simulink model "ISStelerobotics"  (R2022b)
settings: Solver=VariableStepAuto  StartTime=0.0  StopTime=10  RelTol=1e-3
InitFcn:
  | gammaM = [1 0 0; 0 1 0; 0 0 1];
  | gammaS = [1 0 0; 0 1 0; 0 0 1];
  | Km = 300.*[1 0 0; 0 1 0; 0 0 1];
  | Ks = 300.*[1 0 0; 0 1 0; 0 0 1];
settings Model: Creator=negin  LastModifiedBy=Administrator
settings DebuggingCC: UnconnectedInputMsg=warning  UnconnectedOutputMsg=warning  UnconnectedLineMsg=warning
settings ModelReferenceCC: EnableRefExpFcnMdlSchedulingChecks=on
settings RTWCC: DLArmComputeVersion=19.05

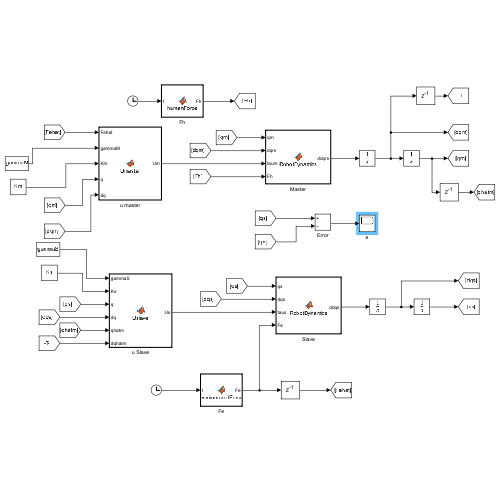
[thumbnail: Simulink's stored preview of the top-level diagram]
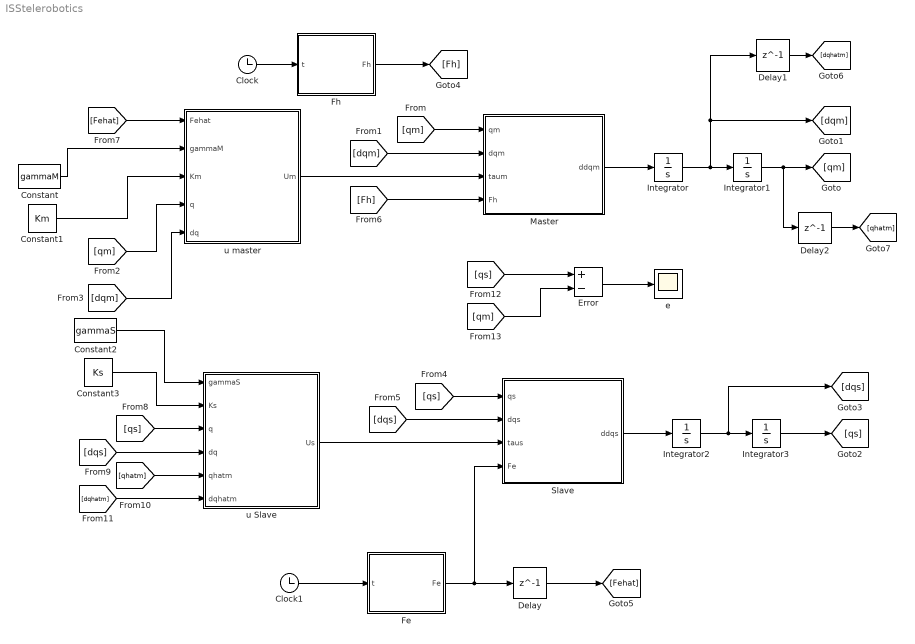
== system ISStelerobotics ==
  Clock : Clock
  Clock1 : Clock
  Constant : Constant  Value=gammaM  VectorParams1D=off
  Constant1 : Constant  Value=Km  VectorParams1D=off
  Constant2 : Constant  Value=gammaS  VectorParams1D=off
  Constant3 : Constant  Value=Ks  VectorParams1D=off
  Delay : Delay  DelayLength=1  InitialCondition=0
  Delay1 : Delay  DelayLength=1  InitialCondition=0
  Delay2 : Delay  DelayLength=1  InitialCondition=0
  Error : Sum  Inputs=+-
  Fe : MATLAB Function  TreatAsAtomicUnit=on
  Fh : MATLAB Function  TreatAsAtomicUnit=on
  Integrator{,1..3} (4 alike) : Integrator  InitialCondition=[0; 0; 0]
  Master : MATLAB Function  TreatAsAtomicUnit=on
  Slave : MATLAB Function  TreatAsAtomicUnit=on
  e : Scope
  u Slave : MATLAB Function  TreatAsAtomicUnit=on
  u master : MATLAB Function  TreatAsAtomicUnit=on
  wires:
  Clock/1 -> Fh/1(t)
  Fh/1(Fh) -> [Fh]
  u master/1(Um) -> Master/3(taum)
  Master/1(ddqm) -> Integrator/1
  Integrator/1 -> Delay1/1, [dqm], Integrator1/1
  Integrator1/1 -> Delay2/1, [qm]
  [qm] -> Master/1(qm)
  [dqm] -> Master/2(dqm)
  Constant/1 -> u master/2(gammaM)
  Constant1/1 -> u master/3(Km)
  [qm] -> u master/4(q)
  [dqm] -> u master/5(dq)
  Slave/1(ddqs) -> Integrator2/1
  Integrator2/1 -> [dqs], Integrator3/1
  Integrator3/1 -> [qs]
  [dqs] -> Slave/2(dqs)
  [qs] -> Slave/1(qs)
  u Slave/1(Us) -> Slave/3(taus)
  [Fh] -> Master/4(Fh)
  Clock1/1 -> Fe/1(t)
  Fe/1(Fe) -> Delay/1, Slave/4(Fe)
  Delay/1 -> [Fehat]
  [Fehat] -> u master/1(Fehat)
  Constant2/1 -> u Slave/1(gammaS)
  Constant3/1 -> u Slave/2(Ks)
  [qs] -> u Slave/3(q)
  [dqs] -> u Slave/4(dq)
  [dqhatm] -> u Slave/6(dqhatm)
  [qhatm] -> u Slave/5(qhatm)
  Delay1/1 -> [dqhatm]
  Delay2/1 -> [qhatm]
  [qs] -> Error/1
  [qm] -> Error/2
  Error/1 -> e/1

== matlab function ISStelerobotics/Master ==
  data: qm input; ddqm output; dqm input; taum input; Fh input
function ddqm = RobotDynamics(qm, dqm, taum, Fh)

m1 = 1;
m2 = 1;
m3 = 1;

l1 = 1;
l2 = 1;
l3 = 1;

r1 = l1/2;
r2 = l2/2;
r3 = l3/2;

R1 = 0.05;
R2 = 0.05;
R3 = 0.05;

g = 9.81;

a1 = m2*r2^2 + m3*l2^2;
a2 = m3*r3^2;
a3 = m3*r3*l2;
b1 = (m2*r2 + m3*l2)*g;
b2 = m3*r3*g;
I1 = 0.5*m1*R1^2;
I2 = 0.5*m2*R2^2;
I3 = 0.5*m3*R3^2;

M11 = a1*cos(qm(2))^2 + a2*cos(qm(2) + qm(3))^2 + 2*a3*cos(qm(2))*cos(qm(2) + qm(3)) + I1;
M12 = 0; 
M13 = 0; 
M21 = 0; 
M31 = 0;
M22 = a1 + a2 + 2*a3*cos(qm(3)) + I2;
M23 = a2 + a3*cos(qm(3));
M32 = a2 + a3*cos(qm(3));
M33 = a2 + I3;
M = [M11 M12 M13; M21 M22 M23; M31 M32 M33];

C11 = -0.5*a1*dqm(2)*sin(2*qm(2)) - 0.5*a2*(dqm(2) + dqm(3))*sin(2*qm(2) + 2*qm(3))...
    - a3*dqm(2)*sin(2*qm(2) + qm(3)) - a3*dqm(3)*cos(qm(2))*sin(qm(2) + qm(3));
C12 = -0.5*a1*dqm(1)*sin(2*qm(2)) - 0.5*a2*dqm(1)*sin(2*qm(2) + 2*qm(3)) - ...
    a3*dqm(1)*sin(2*qm(2) + qm(3));
C13 = -0.5*a2*dqm(1)*sin(2*qm(2) + 2*qm(3)) - a3*dqm(1)*cos(qm(2))*sin(qm(2) + qm(3));
C21 = -C12;
C22 = -a3*dqm(3)*sin(qm(3));
C23 = -a3*(dqm(2) + dqm(3))*sin(qm(3));
C31 = -C13;
C32 = a3*dqm(2)*sin(qm(3));
C33 = 0;
C = [C11 C12 C13; C21 C22 C23; C31 C32 C33];

G11 = 0;
G21 = m2*l2*sin(qm(2))*g/2 - m3*l3*sin(qm(2) + qm(3))*g/2 - m3*l2*sin(qm(2))*g;
G31 = -m3*l3*sin(qm(2) + qm(3))*g/2;
G = [G11; G21; G31];

ddqm = inv(M)*(taum + Fh - C*dqm - G);
end

== matlab function ISStelerobotics/Fh ==
  data: t input; Fh output
function Fh = humanForce(t)

Fh = [t; 2*t; 3*t];

end

== matlab function ISStelerobotics/u master ==
  data: Fehat input; Um output; gammaM input; Km input; q input; dq input
function Um = Umaster(Fehat, gammaM, Km, q, dq)

m1 = 1;
m2 = 1;
m3 = 1;

l1 = 1;
l2 = 1;
l3 = 1;

r1 = l1/2;
r2 = l2/2;
r3 = l3/2;

R1 = 0.05;
R2 = 0.05;
R3 = 0.05;

g = 9.81;

a1 = m2*r2^2 + m3*l2^2;
a2 = m3*r3^2;
a3 = m3*r3*l2;
b1 = (m2*r2 + m3*l2)*g;
b2 = m3*r3*g;
I1 = 0.5*m1*R1^2;
I2 = 0.5*m2*R2^2;
I3 = 0.5*m3*R3^2;

M11 = a1*cos(q(2))^2 + a2*cos(q(2) + q(3))^2 + 2*a3*cos(q(2))*cos(q(2) + q(3)) + I1;
M12 = 0; 
M13 = 0; 
M21 = 0; 
M31 = 0;
M22 = a1 + a2 + 2*a3*cos(q(3)) + I2;
M23 = a2 + a3*cos(q(3));
M32 = a2 + a3*cos(q(3));
M33 = a2 + I3;
M = [M11 M12 M13; M21 M22 M23; M31 M32 M33];

C11 = -0.5*a1*dq(2)*sin(2*q(2)) - 0.5*a2*(dq(2) + dq(3))*sin(2*q(2) + 2*q(3))...
    - a3*dq(2)*sin(2*q(2) + q(3)) - a3*dq(3)*cos(q(2))*sin(q(2) + q(3));
C12 = -0.5*a1*dq(1)*sin(2*q(2)) - 0.5*a2*dq(1)*sin(2*q(2) + 2*q(3)) - ...
    a3*dq(1)*sin(2*q(2) + q(3));
C13 = -0.5*a2*dq(1)*sin(2*q(2) + 2*q(3)) - a3*dq(1)*cos(q(2))*sin(q(2) + q(3));
C21 = -C12;
C22 = -a3*dq(3)*sin(q(3));
C23 = -a3*(dq(2) + dq(3))*sin(q(3));
C31 = -C13;
C32 = a3*dq(2)*sin(q(3));
C33 = 0;
C = [C11 C12 C13; C21 C22 C23; C31 C32 C33];

G11 = 0;
G21 = m2*l2*sin(q(2))*g/2 - m3*l3*sin(q(2) + q(3))*g/2 - m3*l2*sin(q(2))*g;
G31 = -m3*l3*sin(q(2) + q(3))*g/2;
G = [G11; G21; G31];

Um = -M*gammaM*dq - C*gammaM*q + G - Km*(dq + gammaM*q) + Fehat;

end

== matlab function ISStelerobotics/Slave ==
  data: qs input; ddqs output; dqs input; taus input; Fe input
function ddqs = RobotDynamics(qs, dqs, taus, Fe)

m1 = 1;
m2 = 1;
m3 = 1;

l1 = 1;
l2 = 1;
l3 = 1;

r1 = l1/2;
r2 = l2/2;
r3 = l3/2;

R1 = 0.05;
R2 = 0.05;
R3 = 0.05;

g = 9.81;

a1 = m2*r2^2 + m3*l2^2;
a2 = m3*r3^2;
a3 = m3*r3*l2;
b1 = (m2*r2 + m3*l2)*g;
b2 = m3*r3*g;
I1 = 0.5*m1*R1^2;
I2 = 0.5*m2*R2^2;
I3 = 0.5*m3*R3^2;

M11 = a1*cos(qs(2))^2 + a2*cos(qs(2) + qs(3))^2 + 2*a3*cos(qs(2))*cos(qs(2) + qs(3)) + I1;
M12 = 0; 
M13 = 0; 
M21 = 0; 
M31 = 0;
M22 = a1 + a2 + 2*a3*cos(qs(3)) + I2;
M23 = a2 + a3*cos(qs(3));
M32 = a2 + a3*cos(qs(3));
M33 = a2 + I3;
M = [M11 M12 M13; M21 M22 M23; M31 M32 M33];

C11 = -0.5*a1*dqs(2)*sin(2*qs(2)) - 0.5*a2*(dqs(2) + dqs(3))*sin(2*qs(2) + 2*qs(3))...
    - a3*dqs(2)*sin(2*qs(2) + qs(3)) - a3*dqs(3)*cos(qs(2))*sin(qs(2) + qs(3));
C12 = -0.5*a1*dqs(1)*sin(2*qs(2)) - 0.5*a2*dqs(1)*sin(2*qs(2) + 2*qs(3)) - ...
    a3*dqs(1)*sin(2*qs(2) + qs(3));
C13 = -0.5*a2*dqs(1)*sin(2*qs(2) + 2*qs(3)) - a3*dqs(1)*cos(qs(2))*sin(qs(2) + qs(3));
C21 = -C12;
C22 = -a3*dqs(3)*sin(qs(3));
C23 = -a3*(dqs(2) + dqs(3))*sin(qs(3));
C31 = -C13;
C32 = a3*dqs(2)*sin(qs(3));
C33 = 0;
C = [C11 C12 C13; C21 C22 C23; C31 C32 C33];

G11 = 0;
G21 = m2*l2*sin(qs(2))*g/2 - m3*l3*sin(qs(2) + qs(3))*g/2 - m3*l2*sin(qs(2))*g;
G31 = -m3*l3*sin(qs(2) + qs(3))*g/2;
G = [G11; G21; G31];

ddqs = inv(M)*(taus + Fe - C*dqs - G);
end

== matlab function ISStelerobotics/u Slave ==
  data: gammaS input; Us output; Ks input; q input; dq input; qhatm input; dqhatm input
function Us = Uslave(gammaS, Ks, q, dq, qhatm, dqhatm)

m1 = 1;
m2 = 1;
m3 = 1;

l1 = 1;
l2 = 1;
l3 = 1;

r1 = l1/2;
r2 = l2/2;
r3 = l3/2;

R1 = 0.05;
R2 = 0.05;
R3 = 0.05;

g = 9.81;

a1 = m2*r2^2 + m3*l2^2;
a2 = m3*r3^2;
a3 = m3*r3*l2;
b1 = (m2*r2 + m3*l2)*g;
b2 = m3*r3*g;
I1 = 0.5*m1*R1^2;
I2 = 0.5*m2*R2^2;
I3 = 0.5*m3*R3^2;

M11 = a1*cos(q(2))^2 + a2*cos(q(2) + q(3))^2 + 2*a3*cos(q(2))*cos(q(2) + q(3)) + I1;
M12 = 0; 
M13 = 0; 
M21 = 0; 
M31 = 0;
M22 = a1 + a2 + 2*a3*cos(q(3)) + I2;
M23 = a2 + a3*cos(q(3));
M32 = a2 + a3*cos(q(3));
M33 = a2 + I3;
M = [M11 M12 M13; M21 M22 M23; M31 M32 M33];

C11 = -0.5*a1*dq(2)*sin(2*q(2)) - 0.5*a2*(dq(2) + dq(3))*sin(2*q(2) + 2*q(3))...
    - a3*dq(2)*sin(2*q(2) + q(3)) - a3*dq(3)*cos(q(2))*sin(q(2) + q(3));
C12 = -0.5*a1*dq(1)*sin(2*q(2)) - 0.5*a2*dq(1)*sin(2*q(2) + 2*q(3)) - ...
    a3*dq(1)*sin(2*q(2) + q(3));
C13 = -0.5*a2*dq(1)*sin(2*q(2) + 2*q(3)) - a3*dq(1)*cos(q(2))*sin(q(2) + q(3));
C21 = -C12;
C22 = -a3*dq(3)*sin(q(3));
C23 = -a3*(dq(2) + dq(3))*sin(q(3));
C31 = -C13;
C32 = a3*dq(2)*sin(q(3));
C33 = 0;
C = [C11 C12 C13; C21 C22 C23; C31 C32 C33];

G11 = 0;
G21 = m2*l2*sin(q(2))*g/2 - m3*l3*sin(q(2) + q(3))*g/2 - m3*l2*sin(q(2))*g;
G31 = -m3*l3*sin(q(2) + q(3))*g/2;
G = [G11; G21; G31];

Us = M*gammaS*(dqhatm - dq) + C*gammaS*(qhatm - q) + G - Ks*(dq + gammaS*(q - qhatm));

end

== matlab function ISStelerobotics/Fe ==
  data: t input; Fe output
function Fe = environmentForce(t)

Fe = [0.5*t; 0.6*t; 0.7*t];

end
